simulink model "sample14"  (R2019a)
settings: Solver=VariableStepAuto  StartTime=0.0  StopTime=10.0  RelTol=1e-3
settings Model: Creator=welcome  LastModifiedBy=welcome

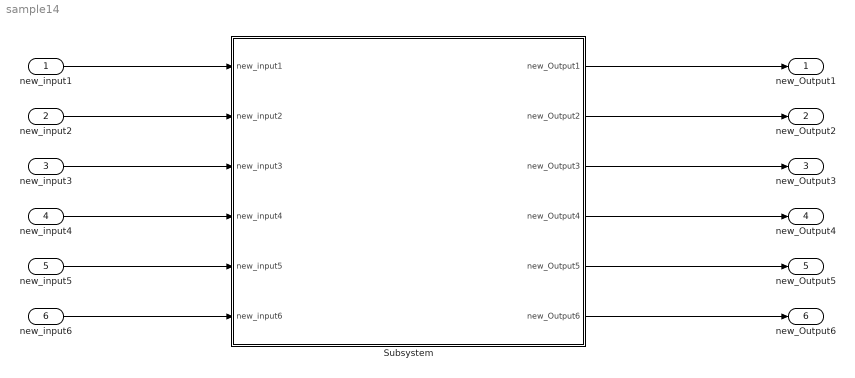
== system sample14 ==
  new_input1 : Inport
  new_input2 : Inport  Port=2
  new_input3 : Inport  Port=3
  new_input4 : Inport  Port=4
  new_input5 : Inport  Port=5
  new_input6 : Inport  Port=6
  Subsystem : Subsystem
  new_Output1 : Outport
  new_Output2 : Outport  Port=2
  new_Output3 : Outport  Port=3
  new_Output4 : Outport  Port=4
  new_Output5 : Outport  Port=5
  new_Output6 : Outport  Port=6
  wires:
  new_input1/1 -> Subsystem/1(new_input1)
  new_input2/1 -> Subsystem/2(new_input2)
  new_input3/1 -> Subsystem/3(new_input3)
  new_input4/1 -> Subsystem/4(new_input4)
  new_input5/1 -> Subsystem/5(new_input5)
  new_input6/1 -> Subsystem/6(new_input6)
  Subsystem/1(new_Output1) -> new_Output1/1
  Subsystem/2(new_Output2) -> new_Output2/1
  Subsystem/3(new_Output3) -> new_Output3/1
  Subsystem/4(new_Output4) -> new_Output4/1
  Subsystem/5(new_Output5) -> new_Output5/1
  Subsystem/6(new_Output6) -> new_Output6/1

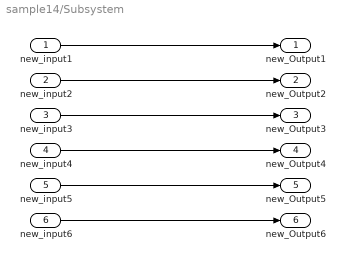
== system sample14/Subsystem ==
  new_input1 : Inport
  new_input2 : Inport  Port=2
  new_input3 : Inport  Port=3
  new_input4 : Inport  Port=4
  new_input5 : Inport  Port=5
  new_input6 : Inport  Port=6
  new_Output1 : Outport
  new_Output2 : Outport  Port=2
  new_Output3 : Outport  Port=3
  new_Output4 : Outport  Port=4
  new_Output5 : Outport  Port=5
  new_Output6 : Outport  Port=6
  wires:
  new_input1/1 -> new_Output1/1
  new_input2/1 -> new_Output2/1
  new_input3/1 -> new_Output3/1
  new_input4/1 -> new_Output4/1
  new_input5/1 -> new_Output5/1
  new_input6/1 -> new_Output6/1
